simulink model "flightControlSystem"  (R2021a)
settings: Solver=ode3  StartTime=0  StopTime=TFinal  FixedStep=Ts  RelTol=1e-3  EnableMultiTasking=on
undefined symbols (not defined in the file): BINARIZATION_THRESHOLD, CENTER_THRESHOLD, codertarget, COG_X, COG_Y, Controller, DELAY_LANDING, DERIVATIVE_GAIN, DiscIntNeverNeededParam, Discrete, DISK_KERNEL, Estimator, FLAG_WAIT_FOR_HOVERING, FRAME_SIZE_HEIGHT, FRAME_SIZE_WIDTH, g, G_B_GAIN, GAIN_LANDING, GAIN_TRACK, init, Sensors, strel, Time, TIME_HOLD, Ts, var_acc_angle_N, var_bias_gyr_N, var_gyro_p_N, Vehicle, Z_HIGH, Z_LOW
libraries: simulink x39, ctrlSharedLib x4, sharedtransform x3, visionmorphops x1, parrotlib x1
(part 3 of 3)

== stateflow chart flightControlSystem/Control System/Path Planning/Non linear Path Planner/X_PLANNER/Chart1 ==
  state STATE [group]
    - TRACKING: The drone is tracking the lane or the end-marker.
    - LANDING: The drone is landing if the end-marker is detected and the error between the drone CoG and the middle
    point of the end-marker is less than MAX_ERROR_LANDING.
    - TRACK_DETECTED: The Image Processing System detected the lane.
    - END_MARKER_DETECTED: The Image Processing System detected the end-marker.
  state INPUT [group]
    - flag_track: flag raised when the track is detected by the Image Processing System.
    - flag_end_marker_to_controller: flag raised when the drone has to land.
    - lin_part: linear part of the path planner.
    - dev_part: derivative part of the path planner.
    - x_estimated: postion x estimated from the sensors.
    - flag_end_marker: flag raised when the land-marker is detected by the Image Processing System.
  state OUTPUT [group]
    - x_planned: x coordinate of the goal position.
  state LANDING
    during:
    x_planned=x_planned_stored;
  state TRACK_MARKER
    during:
    x_planned = x_estimated + 0.05;
  state END_MARKER_DETECTED
    entry:
    circle_count = circle_count + 1;
    during:
    x_planned = x_estimated + lin_part ;
    x_planned_stored = x_planned;
  state TAKE_OFF
    x_planned = 0;
  state TRACK_MARKER2
    during:
    x_planned = x_estimated + 0.1;
  (default) -> TAKE_OFF : {circle_count = 0}
  TRACK_MARKER -> END_MARKER_DETECTED : [ flag_end_marker==1 && flag_track==0]
  TAKE_OFF -> TRACK_MARKER : [after(5,sec)]
  END_MARKER_DETECTED -> LANDING : [flag_end_marker_to_controller==1]
  TRACK_MARKER2 -> TRACK_MARKER : [flag_end_marker == 0]
  LANDING -> TRACK_MARKER2 : [flag_hover == 1 && circle_count <= 1]
  data: dev_part input double; lin_part input double; x_planned output double; flag_end_marker_to_controller input double; x_estimated input double; flag_track input double; x_planned_stored local double; flag_end_marker input double; circle_count local double; flag_hover input
